simulink model "all_topologies"  (R2016a)
settings: Solver=ode4  StartTime=0.0  StopTime=stop_time  FixedStep=Sampling_time  RelTol=1e-3
values from neighbouring files (symbols this model uses):
  DCLINK_Cap = capacitorselection(Is,ma,pf,ns,np,sw_frequency,Vdc,Pout,Lsm,Efm)    [alltopologies.m]    (also in capacitorselection.m = Cdcreq)
  Ef = Efm    [capacitorselection.m]    (also in loadsourcesettings.m = 154.55)
  intangle1 = 0    [loadsourcesettings.m]
  intangle2 = intangle1 + interleaving_angle    [loadsourcesettings.m]
  intangle3 = intangle1    (= 0)    [loadsourcesettings.m]
  intangle4 = intangle2    [loadsourcesettings.m]
  Load_Angle = delta*pi/180    [loadsourcesettings.m]
  Ls = Lsm    [capacitorselection.m]    (also in loadsourcesettings.m = 0.0276)
  ma = 0.9    [alltopologies.m]    (also in loadsourcesettings.m = (Vtll)/(Vdcm*0.612))
  ref_frequency = 2*pi*50    (= 314.159265359)    [alltopologies.m]    (also in loadsourcesettings.m)
  Sampling_time = 1e-6    (= 1e-06)    [alltopologies.m]
  Vin = Vdc + Rin*(Pout/Vdc)    [capacitorselection.m]    (also in loadsourcesettings.m)
undefined symbols (not defined in the file or in its folder): DCLINK_Cap2, Rload
libraries: powerlib x172, powerlib_meascontrol x95, simulink x24
(part 2 of 2)

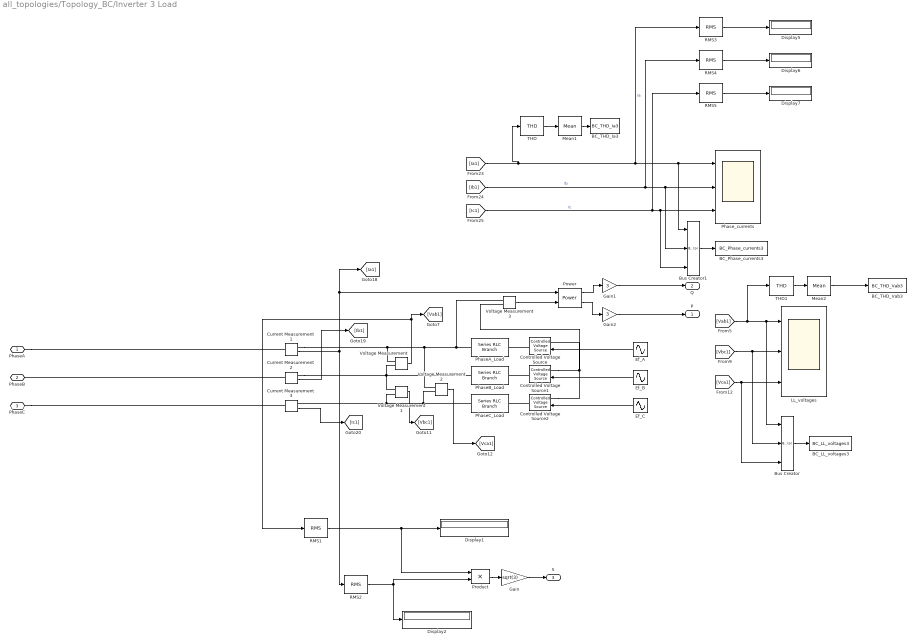
== system all_topologies/Topology_BC/Inverter 3 Load ==
  BC_LL_voltages3 : ToWorkspace  VariableName=BC_LL_voltages3  SaveFormat=Structure With Time  SampleTime=-1
  BC_Phase_currents3 : ToWorkspace  VariableName=BC_Phase_currents3  SaveFormat=Structure With Time  SampleTime=-1
  BC_THD_Ia3 : ToWorkspace  VariableName=BC_THD_Ia3  SaveFormat=Structure With Time  SampleTime=-1
  BC_THD_Vab3 : ToWorkspace  VariableName=BC_THD_Vab3  SaveFormat=Structure With Time  SampleTime=-1
  Bus Creator : BusCreator  Inputs=3
  Bus Creator1 : BusCreator  Inputs=3
  Controlled Voltage Source : powerlib/Electrical Sources/Controlled Voltage Source  Initialize=on  Source_Type=AC  Amplitude=0  Phase=0  Frequency=0  Measurements=None
  Controlled Voltage Source1 : powerlib/Electrical Sources/Controlled Voltage Source  Initialize=on  Source_Type=AC  Amplitude=0  Phase=0  Frequency=0  Measurements=None
  Controlled Voltage Source2 : powerlib/Electrical Sources/Controlled Voltage Source  Initialize=on  Source_Type=AC  Amplitude=0  Phase=0  Frequency=0  Measurements=None
  Current Measurement1 : powerlib/Measurements/Current Measurement  PhasorSimulation=off  OutputType=Complex  PSBequivalent=0
  Current Measurement2 : powerlib/Measurements/Current Measurement  PhasorSimulation=off  OutputType=Complex  PSBequivalent=0
  Current Measurement3 : powerlib/Measurements/Current Measurement  PhasorSimulation=off  OutputType=Complex  PSBequivalent=0
  Display{1..2,5..7} (5 alike) : Display
  Ef_A : Sin  Amplitude=Ef*sqrt(2)  Frequency=ref_frequency  SampleTime=0
  Ef_B : Sin  Amplitude=Ef*sqrt(2)  Frequency=ref_frequency  Phase=-2*pi/3  SampleTime=0
  Ef_C : Sin  Amplitude=Ef*sqrt(2)  Frequency=ref_frequency  Phase=2*pi/3  SampleTime=0
  Gain : Gain  Gain=sqrt(3)
  Gain1 : Gain  Gain=3
  Gain2 : Gain  Gain=3
  LL_voltages : Scope  NumInputPorts=3
  Mean1 : powerlib_meascontrol/Measurements/Mean  Freq=THD_mean_frequency  Vinit=0  Ts=0
  Mean2 : powerlib_meascontrol/Measurements/Mean  Freq=THD_mean_frequency  Vinit=0  Ts=0
  PhaseA_Load : powerlib/Elements/Series RLC Branch  LConnTagsString=__new0  RConnTagsString=__new0  BranchType=L  Resistance=Rload  Inductance=Ls  SetiL0=off  InitialCurrent=0  Capacitance=1e-6  Setx0=off  InitialVoltage=0  Measurements=None
  PhaseB_Load : powerlib/Elements/Series RLC Branch  LConnTagsString=__new0  RConnTagsString=__new0  BranchType=L  Resistance=Rload  Inductance=Ls  SetiL0=off  InitialCurrent=0  Capacitance=1e-6  Setx0=off  InitialVoltage=0  Measurements=None
  PhaseC_Load : powerlib/Elements/Series RLC Branch  LConnTagsString=__new0  RConnTagsString=__new0  BranchType=L  Resistance=Rload  Inductance=Ls  SetiL0=off  InitialCurrent=0  Capacitance=1e-6  Setx0=off  InitialVoltage=0  Measurements=None
  Phase_currents : Scope  NumInputPorts=3
  Power : powerlib_meascontrol/Measurements/Power  Freq=50  Vinit=[1, 0]  Iinit=[1, 0]  Ts=0
  Product : Product
  RMS1 : powerlib_meascontrol/Measurements/RMS  TrueRMS=off  Freq=Load_Nominal_Freq  RMSInit=120  Ts=0
  RMS{2..5} (4 alike) : powerlib_meascontrol/Measurements/RMS  TrueRMS=on  Freq=Load_Nominal_Freq  RMSInit=120  Ts=0
  THD : powerlib_meascontrol/Measurements/THD  Freq=50  Ts=0
  THD1 : powerlib_meascontrol/Measurements/THD  Freq=50  Ts=0
  Voltage Measurement{,1..3} (4 alike) : powerlib/Measurements/Voltage Measurement  PhasorSimulation=off  OutputType=Complex  PSBequivalent=0
  PhaseA : PMIOPort  Port=1  Side=Left
  PhaseB : PMIOPort  Port=2  Side=Left
  PhaseC : PMIOPort  Port=3  Side=Left
  P : Outport
  Q : Outport  Port=2
  S : Outport  Port=3
  wires:
  Current Measurement2/1 -> [Ib1]
  Voltage Measurement/1 -> [Vab1], RMS1/1
  Voltage Measurement1/1 -> [Vbc1]
  Current Measurement3/1 -> [Ic1]
  [Ia1] -> THD/1, RMS3/1, Bus Creator1/1, Phase_currents/1  "Ia"
  [Ic1] -> RMS5/1, Bus Creator1/3, Phase_currents/3  "Ic"
  THD/1 -> Mean1/1
  Voltage Measurement2/1 -> [Vca1]
  [Ib1] -> RMS4/1, Bus Creator1/2, Phase_currents/2  "Ib"
  THD1/1 -> Mean2/1
  Product/1 -> Gain/1
  RMS1/1 -> Product/1, Display1/1
  RMS2/1 -> Product/2, Display2/1
  Gain/1 -> S/1
  Power/2 -> Gain1/1
  Power/1 -> Gain2/1
  Voltage Measurement3/1 -> Power/1
  Gain1/1 -> Q/1
  Gain2/1 -> P/1
  RMS3/1 -> Display5/1
  RMS4/1 -> Display6/1
  RMS5/1 -> Display7/1
  Current Measurement1/1 -> [Ia1], Power/2, RMS2/1
  Ef_A/1 -> Controlled Voltage Source/1
  Ef_B/1 -> Controlled Voltage Source1/1
  Ef_C/1 -> Controlled Voltage Source2/1
  Mean1/1 -> BC_THD_Ia3/1
  Mean2/1 -> BC_THD_Vab3/1
  [Vca1] -> Bus Creator/3, LL_voltages/3
  [Vab1] -> THD1/1, Bus Creator/1, LL_voltages/1
  [Vbc1] -> LL_voltages/2, Bus Creator/2
  Bus Creator/1 -> BC_LL_voltages3/1
  Bus Creator1/1 -> BC_Phase_currents3/1
  connections:
  Current Measurement2/RConn1 -- Voltage Measurement1/LConn1 -- Voltage Measurement/LConn2 -- PhaseB_Load/LConn1
  PhaseC/RConn1 -- Current Measurement3/LConn1
  PhaseC_Load/LConn1 -- Voltage Measurement2/LConn1 -- Voltage Measurement1/LConn2 -- Current Measurement3/RConn1
  Current Measurement2/LConn1 -- PhaseB/RConn1
  PhaseA/RConn1 -- Current Measurement1/LConn1
  Current Measurement1/RConn1 -- Voltage Measurement/LConn1 -- Voltage Measurement2/LConn2 -- Voltage Measurement3/LConn1 -- PhaseA_Load/LConn1
  Controlled Voltage Source2/LConn1 -- Controlled Voltage Source1/LConn1 -- Voltage Measurement3/LConn2 -- Controlled Voltage Source/LConn1
  Controlled Voltage Source1/RConn1 -- PhaseB_Load/RConn1
  Controlled Voltage Source/RConn1 -- PhaseA_Load/RConn1
  Controlled Voltage Source2/RConn1 -- PhaseC_Load/RConn1

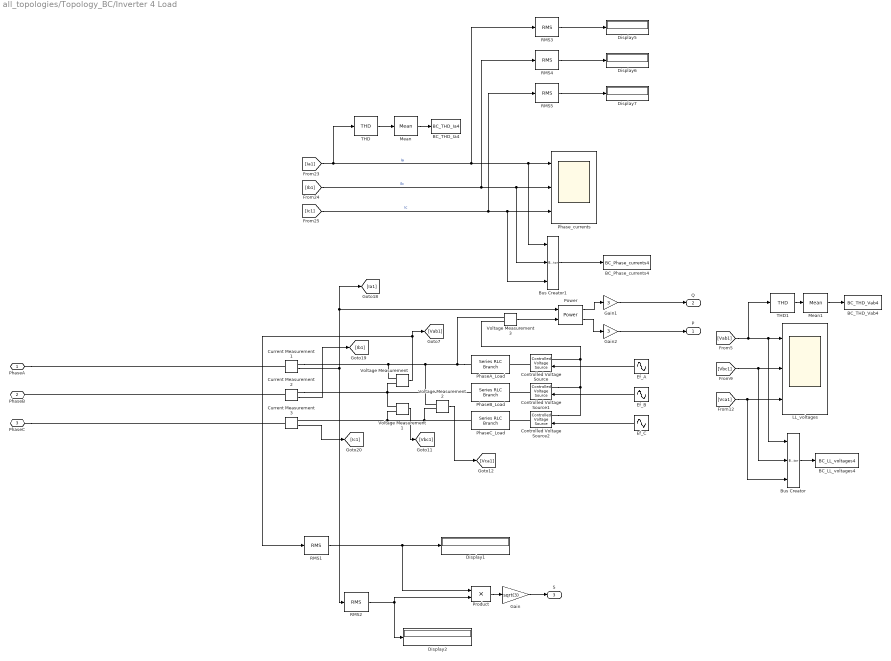
== system all_topologies/Topology_BC/Inverter 4 Load ==
  BC_LL_voltages4 : ToWorkspace  VariableName=BC_LL_voltages4  SaveFormat=Structure With Time  SampleTime=-1
  BC_Phase_currents4 : ToWorkspace  VariableName=BC_Phase_currents4  SaveFormat=Structure With Time  SampleTime=-1
  BC_THD_Ia4 : ToWorkspace  VariableName=BC_THD_Ia4  SaveFormat=Structure With Time  SampleTime=-1
  BC_THD_Vab4 : ToWorkspace  VariableName=BC_THD_Vab4  SaveFormat=Structure With Time  SampleTime=-1
  Bus Creator : BusCreator  Inputs=3
  Bus Creator1 : BusCreator  Inputs=3
  Controlled Voltage Source : powerlib/Electrical Sources/Controlled Voltage Source  Initialize=on  Source_Type=AC  Amplitude=0  Phase=0  Frequency=0  Measurements=None
  Controlled Voltage Source1 : powerlib/Electrical Sources/Controlled Voltage Source  Initialize=on  Source_Type=AC  Amplitude=0  Phase=0  Frequency=0  Measurements=None
  Controlled Voltage Source2 : powerlib/Electrical Sources/Controlled Voltage Source  Initialize=on  Source_Type=AC  Amplitude=0  Phase=0  Frequency=0  Measurements=None
  Current Measurement1 : powerlib/Measurements/Current Measurement  PhasorSimulation=off  OutputType=Complex  PSBequivalent=0
  Current Measurement2 : powerlib/Measurements/Current Measurement  PhasorSimulation=off  OutputType=Complex  PSBequivalent=0
  Current Measurement3 : powerlib/Measurements/Current Measurement  PhasorSimulation=off  OutputType=Complex  PSBequivalent=0
  Display{1..2,5..7} (5 alike) : Display
  Ef_A : Sin  Amplitude=Ef*sqrt(2)  Frequency=ref_frequency  SampleTime=0
  Ef_B : Sin  Amplitude=Ef*sqrt(2)  Frequency=ref_frequency  Phase=-2*pi/3  SampleTime=0
  Ef_C : Sin  Amplitude=Ef*sqrt(2)  Frequency=ref_frequency  Phase=2*pi/3  SampleTime=0
  Gain : Gain  Gain=sqrt(3)
  Gain1 : Gain  Gain=3
  Gain2 : Gain  Gain=3
  LL_voltages : Scope  NumInputPorts=3
  Mean : powerlib_meascontrol/Measurements/Mean  Freq=THD_mean_frequency  Vinit=0  Ts=0
  Mean1 : powerlib_meascontrol/Measurements/Mean  Freq=THD_mean_frequency  Vinit=0  Ts=0
  PhaseA_Load : powerlib/Elements/Series RLC Branch  LConnTagsString=__new0  RConnTagsString=__new0  BranchType=L  Resistance=Rload  Inductance=Ls  SetiL0=off  InitialCurrent=0  Capacitance=1e-6  Setx0=off  InitialVoltage=0  Measurements=None
  PhaseB_Load : powerlib/Elements/Series RLC Branch  LConnTagsString=__new0  RConnTagsString=__new0  BranchType=L  Resistance=Rload  Inductance=Ls  SetiL0=off  InitialCurrent=0  Capacitance=1e-6  Setx0=off  InitialVoltage=0  Measurements=None
  PhaseC_Load : powerlib/Elements/Series RLC Branch  LConnTagsString=__new0  RConnTagsString=__new0  BranchType=L  Resistance=Rload  Inductance=Ls  SetiL0=off  InitialCurrent=0  Capacitance=1e-6  Setx0=off  InitialVoltage=0  Measurements=None
  Phase_currents : Scope  NumInputPorts=3
  Power : powerlib_meascontrol/Measurements/Power  Freq=50  Vinit=[1, 0]  Iinit=[1, 0]  Ts=0
  Product : Product
  RMS1 : powerlib_meascontrol/Measurements/RMS  TrueRMS=off  Freq=Load_Nominal_Freq  RMSInit=120  Ts=0
  RMS{2..5} (4 alike) : powerlib_meascontrol/Measurements/RMS  TrueRMS=on  Freq=Load_Nominal_Freq  RMSInit=120  Ts=0
  THD : powerlib_meascontrol/Measurements/THD  Freq=50  Ts=0
  THD1 : powerlib_meascontrol/Measurements/THD  Freq=50  Ts=0
  Voltage Measurement{,1..3} (4 alike) : powerlib/Measurements/Voltage Measurement  PhasorSimulation=off  OutputType=Complex  PSBequivalent=0
  PhaseA : PMIOPort  Port=1  Side=Left
  PhaseB : PMIOPort  Port=2  Side=Left
  PhaseC : PMIOPort  Port=3  Side=Left
  P : Outport
  Q : Outport  Port=2
  S : Outport  Port=3
  wires:
  Ef_C/1 -> Controlled Voltage Source2/1
  Ef_B/1 -> Controlled Voltage Source1/1
  Ef_A/1 -> Controlled Voltage Source/1
  Current Measurement1/1 -> RMS2/1, Power/2, [Ia1]
  RMS5/1 -> Display7/1
  RMS4/1 -> Display6/1
  RMS3/1 -> Display5/1
  Gain2/1 -> P/1
  Gain1/1 -> Q/1
  Voltage Measurement3/1 -> Power/1
  Power/1 -> Gain2/1
  Power/2 -> Gain1/1
  Gain/1 -> S/1
  RMS2/1 -> Display2/1, Product/2
  RMS1/1 -> Display1/1, Product/1
  Product/1 -> Gain/1
  THD1/1 -> Mean1/1
  [Ib1] -> Bus Creator1/2, Phase_currents/2, RMS4/1  "Ib"
  Voltage Measurement2/1 -> [Vca1]
  [Vca1] -> Bus Creator/3, LL_voltages/3
  [Vab1] -> Bus Creator/1, LL_voltages/1, THD1/1
  [Vbc1] -> Bus Creator/2, LL_voltages/2
  [Ic1] -> Bus Creator1/3, Phase_currents/3, RMS5/1  "Ic"
  [Ia1] -> Bus Creator1/1, Phase_currents/1, RMS3/1, THD/1  "Ia"
  Current Measurement3/1 -> [Ic1]
  Voltage Measurement1/1 -> [Vbc1]
  Voltage Measurement/1 -> RMS1/1, [Vab1]
  Current Measurement2/1 -> [Ib1]
  THD/1 -> Mean/1
  Mean/1 -> BC_THD_Ia4/1
  Mean1/1 -> BC_THD_Vab4/1
  Bus Creator/1 -> BC_LL_voltages4/1
  Bus Creator1/1 -> BC_Phase_currents4/1
  connections:
  Controlled Voltage Source2/RConn1 -- PhaseC_Load/RConn1
  Controlled Voltage Source/RConn1 -- PhaseA_Load/RConn1
  Controlled Voltage Source1/RConn1 -- PhaseB_Load/RConn1
  Controlled Voltage Source/LConn1 -- Voltage Measurement3/LConn2 -- Controlled Voltage Source1/LConn1 -- Controlled Voltage Source2/LConn1
  PhaseA_Load/LConn1 -- Voltage Measurement3/LConn1 -- Voltage Measurement2/LConn2 -- Voltage Measurement/LConn1 -- Current Measurement1/RConn1
  PhaseA/RConn1 -- Current Measurement1/LConn1
  Current Measurement2/LConn1 -- PhaseB/RConn1
  Current Measurement3/RConn1 -- Voltage Measurement1/LConn2 -- Voltage Measurement2/LConn1 -- PhaseC_Load/LConn1
  PhaseC/RConn1 -- Current Measurement3/LConn1
  PhaseB_Load/LConn1 -- Voltage Measurement/LConn2 -- Voltage Measurement1/LConn1 -- Current Measurement2/RConn1

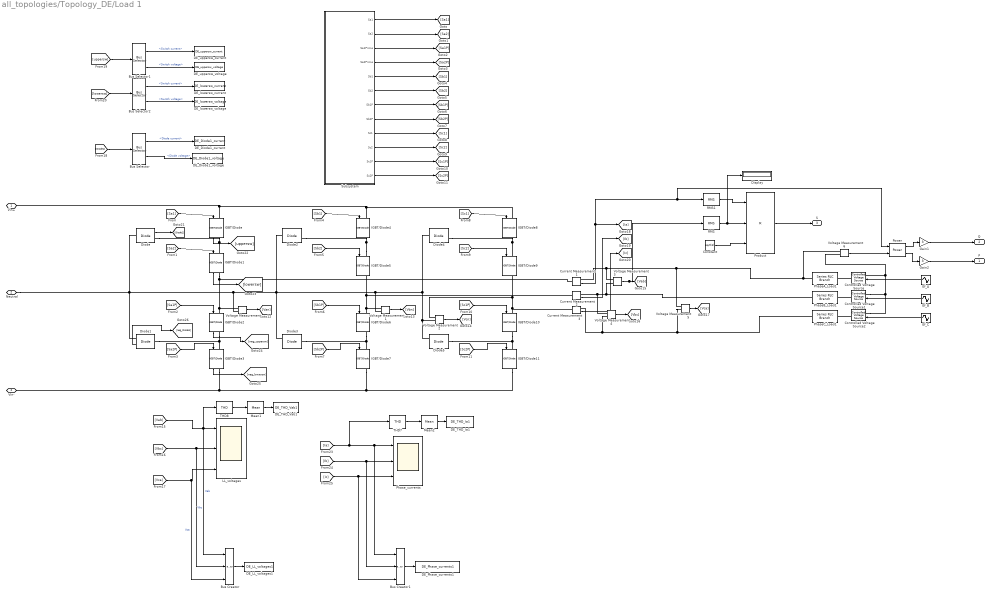
== system all_topologies/Topology_DE/Load 1 ==
  Bus Creator : BusCreator  Inputs=3
  Bus Creator1 : BusCreator  Inputs=3
  Bus Selector : BusSelector  OutputSignals=Diode current,Diode voltage
  Bus Selector1 : BusSelector  OutputSignals=Switch current,Switch voltage
  Bus Selector2 : BusSelector  OutputSignals=Switch current,Switch voltage
  Constant : Constant  Value=sqrt(3)
  Controlled Voltage Source : powerlib/Electrical Sources/Controlled Voltage Source  Initialize=on  Source_Type=AC  Amplitude=0  Phase=0  Frequency=0  Measurements=None
  Controlled Voltage Source1 : powerlib/Electrical Sources/Controlled Voltage Source  Initialize=on  Source_Type=AC  Amplitude=0  Phase=0  Frequency=0  Measurements=None
  Controlled Voltage Source2 : powerlib/Electrical Sources/Controlled Voltage Source  Initialize=on  Source_Type=AC  Amplitude=0  Phase=0  Frequency=0  Measurements=None
  Current Measurement1 : powerlib/Measurements/Current Measurement  PhasorSimulation=off  OutputType=Complex  PSBequivalent=0
  Current Measurement2 : powerlib/Measurements/Current Measurement  PhasorSimulation=off  OutputType=Complex  PSBequivalent=0
  Current Measurement3 : powerlib/Measurements/Current Measurement  PhasorSimulation=off  OutputType=Complex  PSBequivalent=0
  DE_Diode1_current : ToWorkspace  VariableName=DE_Diode1_current  SaveFormat=Structure With Time  SampleTime=-1
  DE_Diode1_voltage : ToWorkspace  VariableName=DE_Diode1_voltage  SaveFormat=Structure With Time  SampleTime=-1
  DE_LL_voltages1 : ToWorkspace  VariableName=DE_LL_voltages1  SaveFormat=Structure With Time  SampleTime=-1
  DE_Phase_currents1 : ToWorkspace  VariableName=DE_Phase_currents1  SaveFormat=Structure With Time  SampleTime=-1
  DE_THD_Ia1 : ToWorkspace  VariableName=DE_THD_Ia1  SaveFormat=Structure With Time  SampleTime=-1
  DE_THD_Vab1 : ToWorkspace  VariableName=DE_THD_Vab1  SaveFormat=Structure With Time  SampleTime=-1
  DE_lowersw_current : ToWorkspace  VariableName=DE_lowersw_current  SaveFormat=Structure With Time  SampleTime=-1
  DE_lowersw_voltage : ToWorkspace  VariableName=DE_lowersw_voltage  SaveFormat=Structure With Time  SampleTime=-1
  DE_uppersw_current : ToWorkspace  VariableName=DE_uppersw_current  SaveFormat=Structure With Time  SampleTime=-1
  DE_uppersw_voltage : ToWorkspace  VariableName=DE_uppersw_voltage  SaveFormat=Structure With Time  SampleTime=-1
  Diode{,1..5} (6 alike) : powerlib/Power Electronics/Diode  Ron=0.001  Lon=0  Vf=0.8  IC=0  UseSnubber=off  Rs=500  Cs=250e-9  Measurements=on
  Display : Display
  Ef_A : Sin  Amplitude=Ef*sqrt(2)  Frequency=ref_frequency  SampleTime=0
  Ef_B : Sin  Amplitude=Ef*sqrt(2)  Frequency=ref_frequency  Phase=-2*pi/3  SampleTime=0
  Ef_C : Sin  Amplitude=Ef*sqrt(2)  Frequency=ref_frequency  Phase=2*pi/3  SampleTime=0
  Gain1 : Gain  Gain=3
  Gain2 : Gain  Gain=3
  IGBT/Diode{,1..11} (12 alike) : powerlib/Power Electronics/IGBT//Diode  Ron=1e-3  Rs=1e5  Cs=inf  Measurements=on
  LL_voltages : Scope  NumInputPorts=3
  Mean1 : powerlib_meascontrol/Measurements/Mean  Freq=THD_mean_frequency  Vinit=0  Ts=0
  Mean2 : powerlib_meascontrol/Measurements/Mean  Freq=THD_mean_frequency  Vinit=0  Ts=0
  PhaseA_Load1 : powerlib/Elements/Series RLC Branch  LConnTagsString=__new0  RConnTagsString=__new0  BranchType=L  Resistance=Rload  Inductance=Ls  SetiL0=off  InitialCurrent=0  Capacitance=1e-6  Setx0=off  InitialVoltage=0  Measurements=None
  PhaseB_Load1 : powerlib/Elements/Series RLC Branch  LConnTagsString=__new0  RConnTagsString=__new0  BranchType=L  Resistance=Rload  Inductance=Ls  SetiL0=off  InitialCurrent=0  Capacitance=1e-6  Setx0=off  InitialVoltage=0  Measurements=None
  PhaseC_Load1 : powerlib/Elements/Series RLC Branch  LConnTagsString=__new0  RConnTagsString=__new0  BranchType=L  Resistance=Rload  Inductance=Ls  SetiL0=off  InitialCurrent=0  Capacitance=1e-6  Setx0=off  InitialVoltage=0  Measurements=None
  Phase_currents : Scope  NumInputPorts=3
  Power : powerlib_meascontrol/Measurements/Power  Freq=50  Vinit=[1, 0]  Iinit=[1, 0]  Ts=0
  Product : Product  Inputs=3
  RMS : powerlib_meascontrol/Measurements/RMS  TrueRMS=off  Freq=50  RMSInit=120  Ts=0
  RMS1 : powerlib_meascontrol/Measurements/RMS  TrueRMS=off  Freq=50  RMSInit=120  Ts=0
  Subsystem : Subsystem
  THD7 : powerlib_meascontrol/Measurements/THD  Freq=Load_Nominal_Freq  Ts=0
  THD8 : powerlib_meascontrol/Measurements/THD  Freq=Load_Nominal_Freq  Ts=0
  Voltage Measurement{,1..6} (7 alike) : powerlib/Measurements/Voltage Measurement  PhasorSimulation=off  OutputType=Complex  PSBequivalent=0
  Vin+ : PMIOPort  Port=1  Side=Left
  Neutral : PMIOPort  Port=2  Side=Left
  Vin- : PMIOPort  Port=3  Side=Left
  P : Outport
  Q : Outport  Port=2
  S : Outport  Port=3
  wires:
  THD7/1 -> Mean2/1
  Diode1/1 -> [neg_Diode1]
  IGBT/Diode3/1 -> [neg_lowersw]
  IGBT/Diode2/1 -> [neg_uppersw]
  Bus Selector2/1 -> DE_lowersw_current/1  "<Switch current>"
  Bus Selector2/2 -> DE_lowersw_voltage/1  "<Switch voltage>"
  Bus Selector1/2 -> DE_uppersw_voltage/1  "<Switch voltage>"
  Bus Selector1/1 -> DE_uppersw_current/1  "<Switch current>"
  [lowersw] -> Bus Selector2/1
  [uppersw] -> Bus Selector1/1
  IGBT/Diode1/1 -> [lowersw]
  IGBT/Diode/1 -> [uppersw]
  Bus Selector/2 -> DE_Diode1_voltage/1  "<Diode voltage>"
  Bus Selector/1 -> DE_Diode1_current/1  "<Diode current>"
  [Diode1] -> Bus Selector/1
  Diode/1 -> [Diode1]
  Current Measurement1/1 -> [Ia], RMS1/1, Power/2
  Voltage Measurement6/1 -> Power/1
  Gain2/1 -> P/1
  Gain1/1 -> Q/1
  Power/1 -> Gain2/1
  Power/2 -> Gain1/1
  Ef_C/1 -> Controlled Voltage Source2/1
  Ef_B/1 -> Controlled Voltage Source1/1
  Ef_A/1 -> Controlled Voltage Source/1
  Product/1 -> S/1
  Constant/1 -> Product/3
  RMS/1 -> Product/2, Display/1
  RMS1/1 -> Product/1
  [Sa1] -> IGBT/Diode/1
  [Sa2] -> IGBT/Diode1/1
  Subsystem/4("Sa2Prime ") -> [Sa2P]
  Subsystem/1("Sa1 ") -> [Sa1]
  Subsystem/2("Sa2 ") -> [Sa2]
  Subsystem/3(Sa1Prime) -> [Sa1P]
  Subsystem/6(Sb2) -> [Sb2]
  [Sa2P] -> IGBT/Diode3/1
  [Sc2P] -> IGBT/Diode11/1
  [Sc1] -> IGBT/Diode8/1
  [Sc1P] -> IGBT/Diode10/1
  Subsystem/8(Sb2P) -> [Sb2P]
  Subsystem/9("Sc1 ") -> [Sc1]
  [Sa1P] -> IGBT/Diode2/1
  Subsystem/12("Sc2P ") -> [Sc2P]
  Voltage Measurement1/1 -> [Vbn]
  [Sb1P] -> IGBT/Diode6/1
  Subsystem/10(Sc2) -> [Sc2]
  Subsystem/11(Sc1P) -> [Sc1P]
  Voltage Measurement2/1 -> [Vcn]
  [Sb2P] -> IGBT/Diode7/1
  [Sb1] -> IGBT/Diode4/1
  [Sc2] -> IGBT/Diode9/1
  Subsystem/5(Sb1) -> [Sb1]
  Subsystem/7("Sb1P ") -> [Sb1P]
  [Sb2] -> IGBT/Diode5/1
  Voltage Measurement/1 -> [Van]
  [Vab] -> THD8/1, Bus Creator/1, LL_voltages/1  "Vab"
  [Vca] -> Bus Creator/3, LL_voltages/3  "Vca"
  [Vbc] -> Bus Creator/2, LL_voltages/2  "Vbc"
  THD8/1 -> Mean1/1
  Current Measurement2/1 -> [Ib]
  Current Measurement3/1 -> [Ic]
  Voltage Measurement3/1 -> [Vab], RMS/1
  Voltage Measurement4/1 -> [Vbc]
  Voltage Measurement5/1 -> [Vca]
  Mean1/1 -> DE_THD_Vab1/1
  Mean2/1 -> DE_THD_Ia1/1
  Bus Creator/1 -> DE_LL_voltages1/1
  [Ib] -> Bus Creator1/2, Phase_currents/2
  [Ia] -> Bus Creator1/1, Phase_currents/1, THD7/1
  [Ic] -> Bus Creator1/3, Phase_currents/3
  Bus Creator1/1 -> DE_Phase_currents1/1
  connections:
  Controlled Voltage Source1/RConn1 -- PhaseB_Load1/RConn1
  Controlled Voltage Source/RConn1 -- PhaseA_Load1/RConn1
  Controlled Voltage Source2/RConn1 -- PhaseC_Load1/RConn1
  Controlled Voltage Source/LConn1 -- Voltage Measurement6/LConn2 -- Controlled Voltage Source2/LConn1 -- Controlled Voltage Source1/LConn1
  IGBT/Diode/RConn1 -- Diode/RConn1 -- IGBT/Diode1/LConn1
  IGBT/Diode8/LConn1 -- IGBT/Diode4/LConn1 -- Vin+/RConn1 -- IGBT/Diode/LConn1
  IGBT/Diode1/RConn1 -- Current Measurement1/LConn1 -- Voltage Measurement/LConn1 -- IGBT/Diode2/LConn1
  IGBT/Diode2/RConn1 -- Diode1/LConn1 -- IGBT/Diode3/LConn1
  Diode5/LConn1 -- IGBT/Diode11/LConn1 -- IGBT/Diode10/RConn1
  IGBT/Diode5/LConn1 -- Diode2/RConn1 -- IGBT/Diode4/RConn1
  Diode4/RConn1 -- IGBT/Diode8/RConn1 -- IGBT/Diode9/LConn1
  IGBT/Diode6/RConn1 -- Diode3/LConn1 -- IGBT/Diode7/LConn1
  IGBT/Diode9/RConn1 -- Voltage Measurement2/LConn1 -- Current Measurement3/LConn1 -- IGBT/Diode10/LConn1
  IGBT/Diode5/RConn1 -- Voltage Measurement1/LConn1 -- IGBT/Diode6/LConn1 -- Current Measurement2/LConn1
  Diode5/RConn1 -- Voltage Measurement2/LConn2 -- Diode4/LConn1 -- Voltage Measurement1/LConn2 -- Diode3/RConn1 -- Voltage Measurement/LConn2 -- Diode1/RConn1 -- Neutral/RConn1 -- Diode/LConn1 -- Diode2/LConn1
  IGBT/Diode11/RConn1 -- Vin-/RConn1 -- IGBT/Diode3/RConn1 -- IGBT/Diode7/RConn1
  Voltage Measurement3/LConn2 -- PhaseB_Load1/LConn1 -- Voltage Measurement4/LConn1 -- Current Measurement2/RConn1
  Voltage Measurement3/LConn1 -- Current Measurement1/RConn1 -- PhaseA_Load1/LConn1 -- Voltage Measurement6/LConn1 -- Voltage Measurement5/LConn2
  Voltage Measurement4/LConn2 -- Current Measurement3/RConn1 -- PhaseC_Load1/LConn1 -- Voltage Measurement5/LConn1

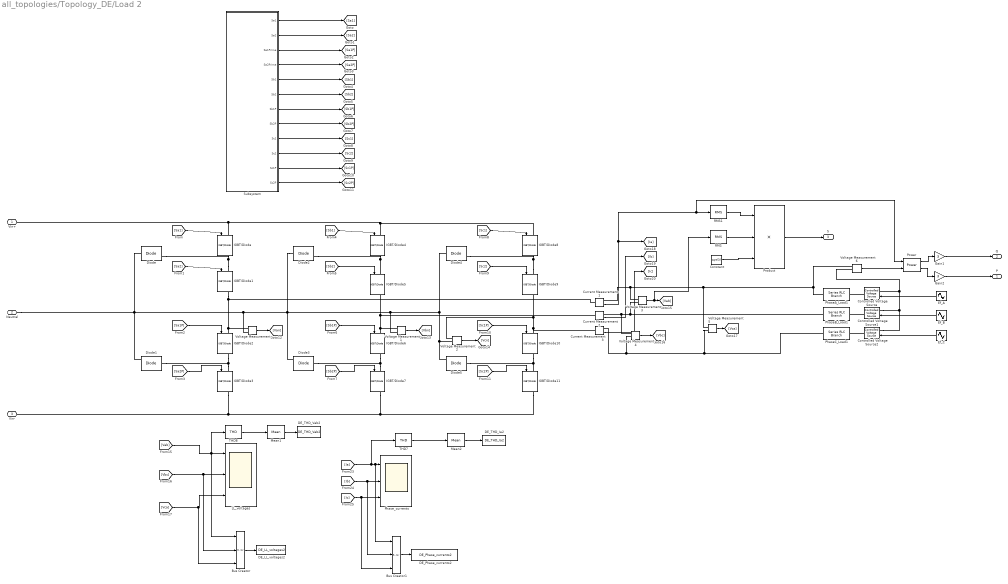
== system all_topologies/Topology_DE/Load 2 ==
  Bus Creator : BusCreator  Inputs=3
  Bus Creator1 : BusCreator  Inputs=3
  Constant : Constant  Value=sqrt(3)
  Controlled Voltage Source : powerlib/Electrical Sources/Controlled Voltage Source  Initialize=on  Source_Type=AC  Amplitude=0  Phase=0  Frequency=0  Measurements=None
  Controlled Voltage Source1 : powerlib/Electrical Sources/Controlled Voltage Source  Initialize=on  Source_Type=AC  Amplitude=0  Phase=0  Frequency=0  Measurements=None
  Controlled Voltage Source2 : powerlib/Electrical Sources/Controlled Voltage Source  Initialize=on  Source_Type=AC  Amplitude=0  Phase=0  Frequency=0  Measurements=None
  Current Measurement1 : powerlib/Measurements/Current Measurement  PhasorSimulation=off  OutputType=Complex  PSBequivalent=0
  Current Measurement2 : powerlib/Measurements/Current Measurement  PhasorSimulation=off  OutputType=Complex  PSBequivalent=0
  Current Measurement3 : powerlib/Measurements/Current Measurement  PhasorSimulation=off  OutputType=Complex  PSBequivalent=0
  DE_LL_voltages2 : ToWorkspace  VariableName=DE_LL_voltages2  SaveFormat=Structure With Time  SampleTime=-1
  DE_Phase_currents2 : ToWorkspace  VariableName=DE_Phase_currents2  SaveFormat=Structure With Time  SampleTime=-1
  DE_THD_Ia2 : ToWorkspace  VariableName=DE_THD_Ia2  SaveFormat=Structure With Time  SampleTime=-1
  DE_THD_Vab2 : ToWorkspace  VariableName=DE_THD_Vab2  SaveFormat=Structure With Time  SampleTime=-1
  Diode{,1..5} (6 alike) : powerlib/Power Electronics/Diode  Ron=0.001  Lon=0  Vf=0.8  IC=0  UseSnubber=off  Rs=500  Cs=250e-9  Measurements=on
  Ef_A : Sin  Amplitude=Ef*sqrt(2)  Frequency=ref_frequency  SampleTime=0
  Ef_B : Sin  Amplitude=Ef*sqrt(2)  Frequency=ref_frequency  Phase=-2*pi/3  SampleTime=0
  Ef_C : Sin  Amplitude=Ef*sqrt(2)  Frequency=ref_frequency  Phase=2*pi/3  SampleTime=0
  Gain1 : Gain  Gain=3
  Gain2 : Gain  Gain=3
  IGBT/Diode{,1..11} (12 alike) : powerlib/Power Electronics/IGBT//Diode  Ron=1e-3  Rs=1e5  Cs=inf  Measurements=on
  LL_voltages : Scope  NumInputPorts=3
  Mean1 : powerlib_meascontrol/Measurements/Mean  Freq=THD_mean_frequency  Vinit=0  Ts=0
  Mean2 : powerlib_meascontrol/Measurements/Mean  Freq=THD_mean_frequency  Vinit=0  Ts=0
  PhaseA_Load1 : powerlib/Elements/Series RLC Branch  LConnTagsString=__new0  RConnTagsString=__new0  BranchType=L  Resistance=Rload  Inductance=Ls  SetiL0=off  InitialCurrent=0  Capacitance=1e-6  Setx0=off  InitialVoltage=0  Measurements=None
  PhaseB_Load1 : powerlib/Elements/Series RLC Branch  LConnTagsString=__new0  RConnTagsString=__new0  BranchType=L  Resistance=Rload  Inductance=Ls  SetiL0=off  InitialCurrent=0  Capacitance=1e-6  Setx0=off  InitialVoltage=0  Measurements=None
  PhaseC_Load1 : powerlib/Elements/Series RLC Branch  LConnTagsString=__new0  RConnTagsString=__new0  BranchType=L  Resistance=Rload  Inductance=Ls  SetiL0=off  InitialCurrent=0  Capacitance=1e-6  Setx0=off  InitialVoltage=0  Measurements=None
  Phase_currents : Scope  NumInputPorts=3
  Power : powerlib_meascontrol/Measurements/Power  Freq=50  Vinit=[1, 0]  Iinit=[1, 0]  Ts=0
  Product : Product  Inputs=3
  RMS : powerlib_meascontrol/Measurements/RMS  TrueRMS=off  Freq=50  RMSInit=120  Ts=0
  RMS1 : powerlib_meascontrol/Measurements/RMS  TrueRMS=off  Freq=50  RMSInit=120  Ts=0
  Subsystem : Subsystem
  THD7 : powerlib_meascontrol/Measurements/THD  Freq=Load_Nominal_Freq  Ts=0
  THD8 : powerlib_meascontrol/Measurements/THD  Freq=Load_Nominal_Freq  Ts=0
  Voltage Measurement{,1..6} (7 alike) : powerlib/Measurements/Voltage Measurement  PhasorSimulation=off  OutputType=Complex  PSBequivalent=0
  Vin+ : PMIOPort  Port=1  Side=Left
  Neutral : PMIOPort  Port=2  Side=Left
  Vin- : PMIOPort  Port=3  Side=Left
  P : Outport
  Q : Outport  Port=2
  S : Outport  Port=3
  wires:
  Voltage Measurement6/1 -> Power/1
  Gain2/1 -> P/1
  Gain1/1 -> Q/1
  Power/1 -> Gain2/1
  Power/2 -> Gain1/1
  Ef_C/1 -> Controlled Voltage Source2/1
  Ef_B/1 -> Controlled Voltage Source1/1
  Ef_A/1 -> Controlled Voltage Source/1
  Product/1 -> S/1
  Constant/1 -> Product/3
  RMS/1 -> Product/2
  RMS1/1 -> Product/1
  Voltage Measurement5/1 -> [Vca]
  Voltage Measurement4/1 -> [Vbc]
  Voltage Measurement3/1 -> [Vab], RMS/1
  Current Measurement3/1 -> [Ic]
  Current Measurement2/1 -> [Ib]
  Current Measurement1/1 -> [Ia], RMS1/1, Power/2
  THD8/1 -> Mean1/1
  THD7/1 -> Mean2/1
  [Vbc] -> Bus Creator/2, LL_voltages/2
  Voltage Measurement/1 -> [Van]
  [Sb2] -> IGBT/Diode5/1
  Subsystem/7("Sb1P ") -> [Sb1P]
  Subsystem/5(Sb1) -> [Sb1]
  [Sc2] -> IGBT/Diode9/1
  [Sb1] -> IGBT/Diode4/1
  [Sb2P] -> IGBT/Diode7/1
  Voltage Measurement2/1 -> [Vcn]
  Subsystem/11(Sc1P) -> [Sc1P]
  Subsystem/10(Sc2) -> [Sc2]
  [Sb1P] -> IGBT/Diode6/1
  Voltage Measurement1/1 -> [Vbn]
  Subsystem/12("Sc2P ") -> [Sc2P]
  [Sa1P] -> IGBT/Diode2/1
  Subsystem/9("Sc1 ") -> [Sc1]
  Subsystem/8(Sb2P) -> [Sb2P]
  [Sc1P] -> IGBT/Diode10/1
  [Sc1] -> IGBT/Diode8/1
  [Sc2P] -> IGBT/Diode11/1
  [Sa2P] -> IGBT/Diode3/1
  Subsystem/6(Sb2) -> [Sb2]
  Subsystem/3(Sa1Prime) -> [Sa1P]
  Subsystem/2("Sa2 ") -> [Sa2]
  Subsystem/1("Sa1 ") -> [Sa1]
  Subsystem/4("Sa2Prime ") -> [Sa2P]
  [Sa2] -> IGBT/Diode1/1
  [Sa1] -> IGBT/Diode/1
  Mean1/1 -> DE_THD_Vab2/1
  Mean2/1 -> DE_THD_Ia2/1
  [Vab] -> Bus Creator/1, THD8/1, LL_voltages/1
  [Vca] -> Bus Creator/3, LL_voltages/3
  Bus Creator/1 -> DE_LL_voltages2/1
  [Ib] -> Bus Creator1/2, Phase_currents/2
  [Ia] -> Bus Creator1/1, Phase_currents/1, THD7/1
  [Ic] -> Bus Creator1/3, Phase_currents/3
  Bus Creator1/1 -> DE_Phase_currents2/1
  connections:
  Controlled Voltage Source1/RConn1 -- PhaseB_Load1/RConn1
  Controlled Voltage Source/RConn1 -- PhaseA_Load1/RConn1
  Controlled Voltage Source2/RConn1 -- PhaseC_Load1/RConn1
  Controlled Voltage Source/LConn1 -- Voltage Measurement6/LConn2 -- Controlled Voltage Source2/LConn1 -- Controlled Voltage Source1/LConn1
  Voltage Measurement5/LConn2 -- Voltage Measurement6/LConn1 -- PhaseA_Load1/LConn1 -- Current Measurement1/RConn1 -- Voltage Measurement3/LConn1
  Voltage Measurement5/LConn1 -- PhaseC_Load1/LConn1 -- Current Measurement3/RConn1 -- Voltage Measurement4/LConn2
  Current Measurement2/RConn1 -- Voltage Measurement4/LConn1 -- PhaseB_Load1/LConn1 -- Voltage Measurement3/LConn2
  IGBT/Diode7/RConn1 -- IGBT/Diode3/RConn1 -- Vin-/RConn1 -- IGBT/Diode11/RConn1
  Diode2/LConn1 -- Diode/LConn1 -- Neutral/RConn1 -- Diode1/RConn1 -- Voltage Measurement/LConn2 -- Diode3/RConn1 -- Voltage Measurement1/LConn2 -- Diode4/LConn1 -- Voltage Measurement2/LConn2 -- Diode5/RConn1
  Current Measurement2/LConn1 -- IGBT/Diode6/LConn1 -- Voltage Measurement1/LConn1 -- IGBT/Diode5/RConn1
  IGBT/Diode10/LConn1 -- Current Measurement3/LConn1 -- Voltage Measurement2/LConn1 -- IGBT/Diode9/RConn1
  IGBT/Diode7/LConn1 -- Diode3/LConn1 -- IGBT/Diode6/RConn1
  IGBT/Diode9/LConn1 -- IGBT/Diode8/RConn1 -- Diode4/RConn1
  IGBT/Diode4/RConn1 -- Diode2/RConn1 -- IGBT/Diode5/LConn1
  IGBT/Diode10/RConn1 -- IGBT/Diode11/LConn1 -- Diode5/LConn1
  IGBT/Diode3/LConn1 -- Diode1/LConn1 -- IGBT/Diode2/RConn1
  IGBT/Diode2/LConn1 -- Voltage Measurement/LConn1 -- Current Measurement1/LConn1 -- IGBT/Diode1/RConn1
  IGBT/Diode/LConn1 -- Vin+/RConn1 -- IGBT/Diode4/LConn1 -- IGBT/Diode8/LConn1
  IGBT/Diode1/LConn1 -- Diode/RConn1 -- IGBT/Diode/RConn1

== system all_topologies/Topology_DE/datacollecter ==
  In1 : Inport
  In2 : Inport  Port=2
  In3 : Inport  Port=3
  In4 : Inport  Port=4
  In5 : Inport  Port=5
  In6 : Inport  Port=6
  In7 : Inport  Port=7
  DE_DCLINK_current : ToWorkspace  VariableName=DE_DCLINK_current  SaveFormat=Structure With Time  SampleTime=-1
  DE_DCLINK_current_rms : ToWorkspace  VariableName=DE_DCLINK_current_rms  SaveFormat=Structure With Time  SampleTime=-1
  DE_DCLINK_voltage : ToWorkspace  VariableName=DE_DCLINK_voltage  SaveFormat=Structure With Time  SampleTime=-1
  DE_DCLINK_voltage_mean : ToWorkspace  VariableName=DE_DCLINK_voltage_mean  SaveFormat=Structure With Time  SampleTime=-1
  DE_Ineutral : ToWorkspace  VariableName=DE_Ineutral  SaveFormat=Structure With Time  SampleTime=-1
  DE_lowerc_current : ToWorkspace  VariableName=DE_lowerc_current  SaveFormat=Structure With Time  SampleTime=-1
  DE_lowerc_current_rms : ToWorkspace  VariableName=DE_lowerc_current_rms  SaveFormat=Structure With Time  SampleTime=-1
  DE_lowerc_voltage : ToWorkspace  VariableName=DE_lowerc_voltage  SaveFormat=Structure With Time  SampleTime=-1
  DE_lowerc_voltage_mean : ToWorkspace  VariableName=DE_lowerc_voltage_mean  SaveFormat=Structure With Time  SampleTime=-1
  DE_upperc_current : ToWorkspace  VariableName=DE_upperc_current  SaveFormat=Structure With Time  SampleTime=-1
  DE_upperc_current_rms : ToWorkspace  VariableName=DE_upperc_current_rms  SaveFormat=Structure With Time  SampleTime=-1
  DE_upperc_voltage : ToWorkspace  VariableName=DE_upperc_voltage  SaveFormat=Structure With Time  SampleTime=-1
  DE_upperc_voltage_mean : ToWorkspace  VariableName=DE_upperc_voltage_mean  SaveFormat=Structure With Time  SampleTime=-1
  Mean{,1..6} (7 alike) : powerlib_meascontrol/Measurements/Mean  Freq=THD_mean_frequency  Vinit=0  Ts=0
  RMS{1..4} (4 alike) : powerlib_meascontrol/Measurements/RMS  TrueRMS=on  Freq=Load_Nominal_Freq  RMSInit=10  Ts=0
  neutral current : Scope
  Ineutral : Outport
  upperc_voltage : Outport  Port=2
  lowerc_voltage : Outport  Port=3
  DCLINK_voltage : Outport  Port=4
  DCLINK_current : Outport  Port=5
  lowerc_current : Outport  Port=6
  upperc_current : Outport  Port=7
  wires:
  Mean3/1 -> DCLINK_current/1
  Mean/1 -> DE_DCLINK_voltage_mean/1, DCLINK_voltage/1
  Mean6/1 -> Ineutral/1
  Mean1/1 -> DE_upperc_voltage_mean/1, upperc_voltage/1
  Mean2/1 -> DE_lowerc_voltage_mean/1, lowerc_voltage/1
  Mean5/1 -> upperc_current/1
  In7/1 -> DE_upperc_current/1, RMS3/1
  Mean4/1 -> lowerc_current/1
  RMS2/1 -> DE_lowerc_current_rms/1, Mean4/1
  RMS4/1 -> DE_DCLINK_current_rms/1, Mean3/1
  In3/1 -> Mean2/1, DE_lowerc_voltage/1
  In5/1 -> RMS4/1, DE_DCLINK_current/1
  In1/1 -> DE_Ineutral/1, RMS1/1, neutral current/1
  RMS1/1 -> Mean6/1
  In4/1 -> Mean/1, DE_DCLINK_voltage/1
  In2/1 -> Mean1/1, DE_upperc_voltage/1
  In6/1 -> RMS2/1, DE_lowerc_current/1
  RMS3/1 -> DE_upperc_current_rms/1, Mean5/1

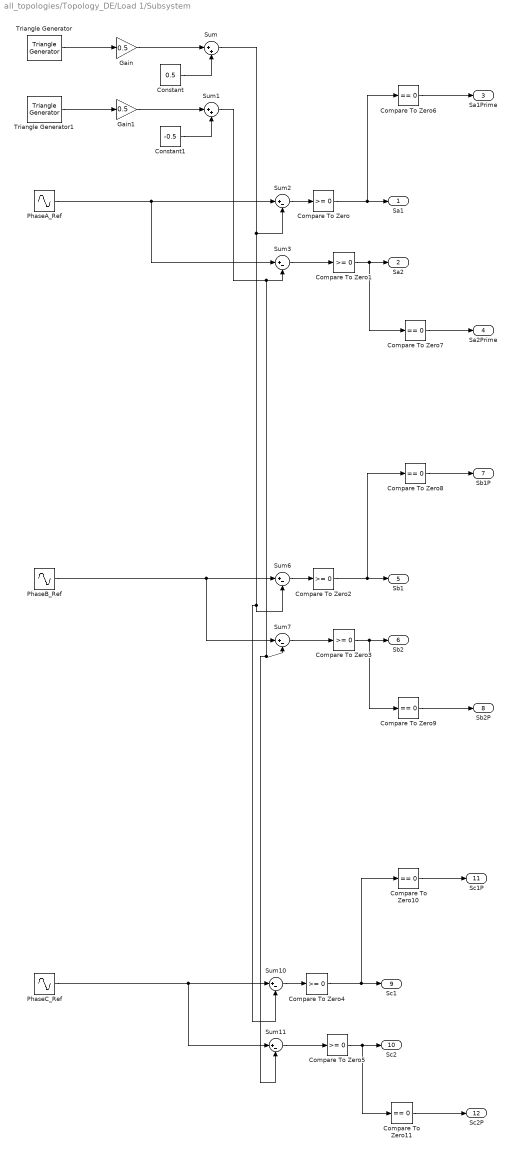
== system all_topologies/Topology_DE/Load 1/Subsystem ==
  Compare To Zero{,1..5} (6 alike) : simulink/Logic and Bit Operations/Compare To Zero  relop=>=  OutDataTypeStr=boolean
  Compare To Zero{6..11} (6 alike) : simulink/Logic and Bit Operations/Compare To Zero  relop===  OutDataTypeStr=boolean
  Constant : Constant  Value=0.5
  Constant1 : Constant  Value=-0.5
  Gain : Gain  Gain=0.5
  Gain1 : Gain  Gain=0.5
  PhaseA_Ref : Sin  Amplitude=ma  Frequency=ref_frequency  Phase=Load_Angle  SampleTime=0
  PhaseB_Ref : Sin  Amplitude=ma  Frequency=ref_frequency  Phase=-2*pi/3+Load_Angle  SampleTime=0
  PhaseC_Ref : Sin  Amplitude=ma  Frequency=ref_frequency  Phase=2*pi/3+Load_Angle  SampleTime=0
  Sum : Sum  Inputs=|++
  Sum1 : Sum  Inputs=|++
  Sum{2..3,6..7,10..11} (6 alike) : Sum  Inputs=|+-
  Triangle Generator : powerlib_meascontrol/Pulse & Signal Generators/Triangle Generator  Freq=sw_frequency  Phase=intangle1  Ts=0
  Triangle Generator1 : powerlib_meascontrol/Pulse & Signal Generators/Triangle Generator  Freq=sw_frequency  Phase=intangle1  Ts=0
  "Sa1 " : Outport
  "Sa2 " : Outport  Port=2
  Sa1Prime : Outport  Port=3
  "Sa2Prime " : Outport  Port=4
  Sb1 : Outport  Port=5
  Sb2 : Outport  Port=6
  "Sb1P " : Outport  Port=7
  Sb2P : Outport  Port=8
  "Sc1 " : Outport  Port=9
  Sc2 : Outport  Port=10
  Sc1P : Outport  Port=11
  "Sc2P " : Outport  Port=12
  wires:
  Triangle Generator/1 -> Gain/1
  Gain/1 -> Sum/1
  Sum/1 -> Sum2/2, Sum10/2, Sum6/2
  Constant/1 -> Sum/2
  Triangle Generator1/1 -> Gain1/1
  Gain1/1 -> Sum1/1
  Sum1/1 -> Sum11/2, Sum7/2, Sum3/2
  Constant1/1 -> Sum1/2
  PhaseA_Ref/1 -> Sum3/1, Sum2/1
  Sum2/1 -> Compare To Zero/1
  Compare To Zero/1 -> Compare To Zero6/1, "Sa1 "/1
  Sum3/1 -> Compare To Zero1/1
  Compare To Zero1/1 -> Compare To Zero7/1, "Sa2 "/1
  Compare To Zero6/1 -> Sa1Prime/1
  Sum6/1 -> Compare To Zero2/1
  Compare To Zero2/1 -> Compare To Zero8/1, Sb1/1
  Sum7/1 -> Compare To Zero3/1
  Compare To Zero3/1 -> Compare To Zero9/1, Sb2/1
  Compare To Zero8/1 -> "Sb1P "/1
  Compare To Zero9/1 -> Sb2P/1
  PhaseB_Ref/1 -> Sum7/1, Sum6/1
  Sum10/1 -> Compare To Zero4/1
  Compare To Zero4/1 -> Compare To Zero10/1, "Sc1 "/1
  Sum11/1 -> Compare To Zero5/1
  Compare To Zero5/1 -> Compare To Zero11/1, Sc2/1
  Compare To Zero10/1 -> Sc1P/1
  Compare To Zero11/1 -> "Sc2P "/1
  PhaseC_Ref/1 -> Sum11/1, Sum10/1
  Compare To Zero7/1 -> "Sa2Prime "/1

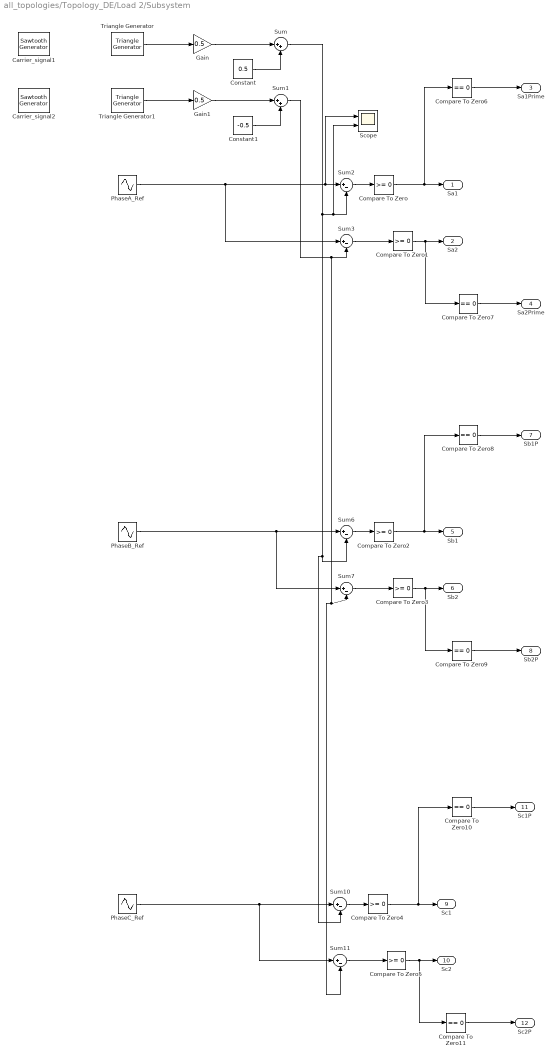
== system all_topologies/Topology_DE/Load 2/Subsystem ==
  Carrier_signal1 : powerlib_meascontrol/Pulse & Signal Generators/Sawtooth Generator  Freq=sw_frequency  Phase=intangle2  Ts=0
  Carrier_signal2 : powerlib_meascontrol/Pulse & Signal Generators/Sawtooth Generator  Freq=sw_frequency  Phase=intangle2  Ts=0
  Compare To Zero{,1..5} (6 alike) : simulink/Logic and Bit Operations/Compare To Zero  relop=>=  OutDataTypeStr=boolean
  Compare To Zero{6..11} (6 alike) : simulink/Logic and Bit Operations/Compare To Zero  relop===  OutDataTypeStr=boolean
  Constant : Constant  Value=0.5
  Constant1 : Constant  Value=-0.5
  Gain : Gain  Gain=0.5
  Gain1 : Gain  Gain=0.5
  PhaseA_Ref : Sin  Amplitude=ma  Frequency=ref_frequency  Phase=Load_Angle  SampleTime=0
  PhaseB_Ref : Sin  Amplitude=ma  Frequency=ref_frequency  Phase=-2*pi/3+Load_Angle  SampleTime=0
  PhaseC_Ref : Sin  Amplitude=ma  Frequency=ref_frequency  Phase=2*pi/3+Load_Angle  SampleTime=0
  Scope : Scope  NumInputPorts=2
  Sum : Sum  Inputs=|++
  Sum1 : Sum  Inputs=|++
  Sum{2..3,6..7,10..11} (6 alike) : Sum  Inputs=|+-
  Triangle Generator : powerlib_meascontrol/Pulse & Signal Generators/Triangle Generator  Freq=sw_frequency  Phase=intangle2  Ts=0
  Triangle Generator1 : powerlib_meascontrol/Pulse & Signal Generators/Triangle Generator  Freq=sw_frequency  Phase=intangle2  Ts=0
  "Sa1 " : Outport
  "Sa2 " : Outport  Port=2
  Sa1Prime : Outport  Port=3
  "Sa2Prime " : Outport  Port=4
  Sb1 : Outport  Port=5
  Sb2 : Outport  Port=6
  "Sb1P " : Outport  Port=7
  Sb2P : Outport  Port=8
  "Sc1 " : Outport  Port=9
  Sc2 : Outport  Port=10
  Sc1P : Outport  Port=11
  "Sc2P " : Outport  Port=12
  wires:
  Compare To Zero7/1 -> "Sa2Prime "/1
  PhaseC_Ref/1 -> Sum10/1, Sum11/1
  Compare To Zero11/1 -> "Sc2P "/1
  Compare To Zero10/1 -> Sc1P/1
  Compare To Zero5/1 -> Sc2/1, Compare To Zero11/1
  Sum11/1 -> Compare To Zero5/1
  Compare To Zero4/1 -> "Sc1 "/1, Compare To Zero10/1
  Sum10/1 -> Compare To Zero4/1
  PhaseB_Ref/1 -> Sum6/1, Sum7/1
  Compare To Zero9/1 -> Sb2P/1
  Compare To Zero8/1 -> "Sb1P "/1
  Compare To Zero3/1 -> Sb2/1, Compare To Zero9/1
  Sum7/1 -> Compare To Zero3/1
  Compare To Zero2/1 -> Sb1/1, Compare To Zero8/1
  Sum6/1 -> Compare To Zero2/1
  Compare To Zero6/1 -> Sa1Prime/1
  Compare To Zero1/1 -> "Sa2 "/1, Compare To Zero7/1
  Sum3/1 -> Compare To Zero1/1
  Compare To Zero/1 -> "Sa1 "/1, Compare To Zero6/1
  Sum2/1 -> Compare To Zero/1
  PhaseA_Ref/1 -> Sum2/1, Scope/1, Sum3/1
  Constant1/1 -> Sum1/2
  Sum1/1 -> Sum3/2, Sum7/2, Sum11/2
  Gain1/1 -> Sum1/1
  Triangle Generator1/1 -> Gain1/1
  Constant/1 -> Sum/2
  Sum/1 -> Sum6/2, Sum10/2, Sum2/2, Scope/2
  Gain/1 -> Sum/1
  Triangle Generator/1 -> Gain/1
